simulink model "Ball_and_beam_sim"  (R2020a)
settings: Solver=VariableStepAuto  StartTime=0.0  StopTime=10.0  RelTol=1e-3
settings Model: Creator=thiag  LastModifiedBy=thiag

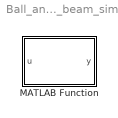
== system Ball_and_beam_sim ==
  MATLAB Function : MATLAB Function  TreatAsAtomicUnit=on

== matlab function Ball_and_beam_sim/MATLAB Function ==
  data: u input; y output
function y = fcn(u)

y = u;
